simulink model "LVI_PDNN_for_QP2"  (R2020b)
settings: Solver=ode15s  StartTime=0.0  StopTime=tEnd  FixedStep=0.  MaxStep=0.2  RelTol=1e-3
values from neighbouring files (symbols this model uses):
  Ann = [-C2;         C2;         -Phi1n;         Phi1n         ]    [CreateNnMatrices.m]    (also in HvsNN.m = [-C2;     C2;     -Phi1n;     Phi1n     ]; MPC_NN.m)
  bnn = [-umin*ones(nc,1) + C1*xk(end);         umax*ones(nc,1) - C1*xk(end);         -ymin*ones(np,1) + Fn*xk + Phi2n*psiPrim;         ymax*ones(np,1) - Fn*xk - Phi2n*psiPrim         ]    [CreateNnMatrices.m]    (also in HvsNN.m = [-umin*ones(nc,1) + C1*xk(end);     umax*ones(nc,1) - C1*xk(; MPC_NN.m)
  eyenn = eye(length(Hnn))    [CreateNnMatrices.m]    (also in HvsNN.m; MPC_NN.m)
  gammann = 10000    [CreateNnMatrices.m]    (also in HvsNN.m = 0.01; MPC_NN.m = 1e+15)
  Hnn = [Wnn  -Ann'; Ann zeros(length(Ann),length(Ann'))]    [CreateNnMatrices.m]    (also in HvsNN.m; MPC_NN.m)
  nc = n_c    (= 5)    [Model_Init_Bayes.m]
  numbConstr = 3*nc + 2*np    [CreateNnMatrices.m]    (also in HvsNN.m; MPC_NN.m)
  pnn = [qnn; -bnn]    [CreateNnMatrices.m]    (also in HvsNN.m; MPC_NN.m)
  qnn = 2*((F*xk)'*W_x*Phi1 + (Phi2*psiPrim)'*W_x*Phi1)'    [CreateNnMatrices.m]    (also in HvsNN.m; MPC_NN.m)
  tEnd = 1e-2    (= 0.01)    [HvsNN.m]    (also in MPC_NN.m = 1e-07)
  Wnn = 2*(Phi1'*W_x*Phi1 + W_u)    [CreateNnMatrices.m]    (also in HvsNN.m; MPC_NN.m)
  xiM = ones(nc,1)*dumin    [CreateNnMatrices.m]    (also in HvsNN.m; MPC_NN.m = ones(nc,1)*dumin.*singleConstraint)
  xiP = ones(nc,1)*dumax    [CreateNnMatrices.m]    (also in HvsNN.m; MPC_NN.m = ones(nc,1)*dumax.*singleConstraint)
  zetaM = [xiM; bigNumber*zeros(length(Ann),1)]    [CreateNnMatrices.m]    (also in HvsNN.m; MPC_NN.m)
  zetaP = [xiP; bigNumber*ones(length(Ann),1)]    [CreateNnMatrices.m]    (also in HvsNN.m; MPC_NN.m)
undefined symbols (not defined in the file or in its folder): DiscIntNeverNeededParam, dnn, Jnn
libraries: simulink x2
settings Model: Creator=Stage  LastModifiedBy=Stage
settings SolverCC: ZeroCrossAlgorithm=Adaptive
settings DebuggingCC: IgnoredZcDiagnostic=none

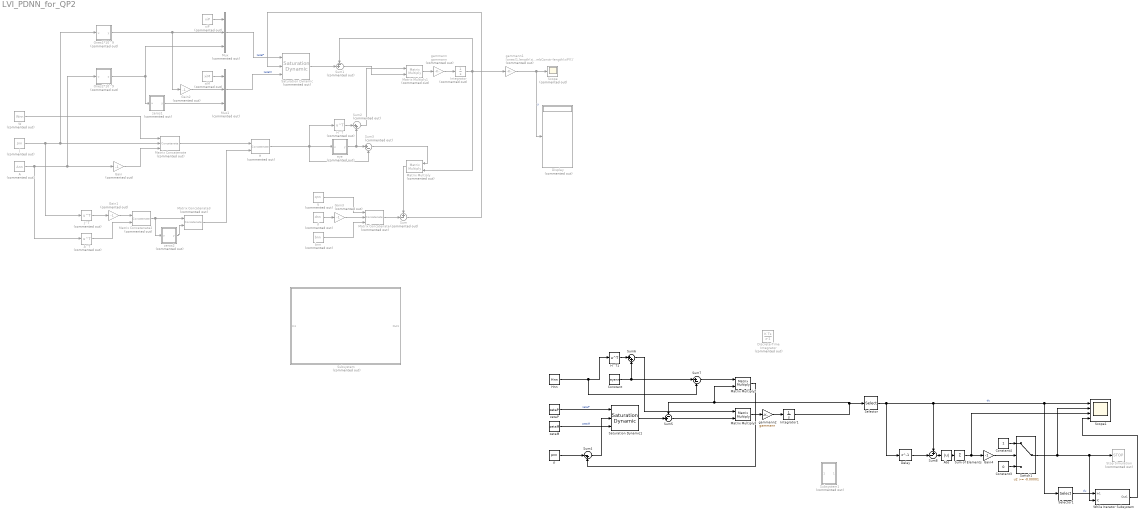
== system LVI_PDNN_for_QP2 ==
  A : Constant  Commented=on  Value=Ann
  A^T : Math  Commented=on  Operator=transpose  SaturateOnIntegerOverflow=on
  Abs : Abs
  Constant : Constant  Value=eyenn
  Constant3 : Constant  Value=0
  Constant4 : Constant
  Delay : Delay  DelayLength=1  SampleTime=tEnd/3
  Discrete-Time Integrator : DiscreteIntegrator  Commented=on  InitialCondition=0.2*(rand(numbConstr,1)-0.5)  SampleTime=0.00000000000001  ICPrevOutput=DiscIntNeverNeededParam  ICPrevScaledInput=DiscIntNeverNeededParam
  Display : Display  Commented=on
  Gain{,1..3} (4 alike) : Gain  Commented=on  Gain=-1
  Gain4 : Gain  Gain=-1
  H : Concatenate  Commented=on  Mode=Multidimensional array  ConcatenateDimension=2
  H^T : Math  Commented=on  Operator=transpose  SaturateOnIntegerOverflow=on
  H^T1 : Math  Operator=transpose  SaturateOnIntegerOverflow=on
  Hnn : Constant  Value=Hnn
  Integrator : Integrator  Commented=on  InitialCondition=0.1*(rand(numbConstr,1)-0.5)*0
  Integrator1 : Integrator  InitialCondition=.10*(rand(numbConstr,1)-0.5)
  J : Constant  Commented=on  Value=Jnn  VectorParams1D=off
  J^T : Math  Commented=on  Operator=transpose  SaturateOnIntegerOverflow=on
  Matrix Concatenate : Concatenate  Commented=on  NumInputs=3  Mode=Multidimensional array
  Matrix Concatenate2 : Concatenate  Commented=on  Mode=Multidimensional array  ConcatenateDimension=2
  Matrix Concatenate3 : Concatenate  Commented=on  Mode=Multidimensional array
  Matrix Concatenate4 : Concatenate  Commented=on  NumInputs=3  Mode=Multidimensional array
  Matrix Multiply : Product  Commented=on  Multiplication=Matrix(*)
  Matrix Multiply1 : Product  Commented=on  Multiplication=Matrix(*)
  Matrix Multiply2 : Product  Multiplication=Matrix(*)
  Matrix Multiply3 : Product  Multiplication=Matrix(*)
  Mux : Mux  Commented=on  Inputs=3
  Mux1 : Mux  Commented=on  Inputs=3
  Ones1*10^9 : MATLAB Function  Commented=on  TreatAsAtomicUnit=on
  Ones2*10^9 : MATLAB Function  Commented=on  TreatAsAtomicUnit=on
  Saturation Dynamic : simulink/Discontinuities/Saturation Dynamic  Commented=on  OutMin=[]  OutMax=[]  OutDataTypeStr=Inherit: Same as second input  OutDataType=fixdt(1, 16)  OutScaling=2^-10  DoSatur=off
  Saturation Dynamic1 : simulink/Discontinuities/Saturation Dynamic  OutMin=[]  OutMax=[]  OutDataTypeStr=Inherit: Same as second input  OutDataType=fixdt(1, 16)  OutScaling=2^-10  DoSatur=off
  Scope : Scope  Commented=on
  Scope1 : Scope  NumInputPorts=4
  Selector : Selector  InputPortWidth=numbConstr  IndexOptions=Index vector (dialog)  Indices=[1:nc]  OutputSizes=1
  Selector1 : Selector  InputPortWidth=nc  IndexOptions=Index vector (dialog)  Indices=[1]  OutputSizes=1
  Stop Simulation : Stop  Commented=on
  Subsystem : Subsystem  Commented=on
  Subsystem1 : Subsystem  Commented=on
  Sum : Sum  Commented=on  Inputs=+-|
  Sum of Elements : Sum  Inputs=+
  Sum1 : Sum  Commented=on  Inputs=-+|
  Sum2 : Sum  Commented=on  Inputs=|++
  Sum3 : Sum  Commented=on  Inputs=|+-
  Sum4 : Sum  Inputs=|-+
  Sum5 : Sum  Inputs=-+|
  Sum6 : Sum  Inputs=|++
  Sum7 : Sum  Inputs=|+-
  Sum8 : Sum  Inputs=+-|
  Switch1 : Switch  Threshold=-0.00001
  W : Constant  Commented=on  Value=Wnn
  While Iterator Subsystem : Subsystem  TreatAsAtomicUnit=on
  bnn : Constant  Commented=on  Value=bnn  VectorParams1D=off
  d : Constant  Commented=on  Value=dnn  VectorParams1D=off
  eye : MATLAB Function  Commented=on  TreatAsAtomicUnit=on
  gammann : Gain  Commented=on  Gain=gammann
  gammann1 : Gain  Commented=on  Gain=[ones(1,length(xiP)) zeros(1,numbConstr-length(xiP))]'
  gammann2 : Gain  Gain=gammann
  p : Constant  Value=pnn  VectorParams1D=off
  q : Constant  Commented=on  Value=qnn  VectorParams1D=off
  xiM : Constant  Commented=on  Value=xiM  VectorParams1D=off
  xiP : Constant  Commented=on  Value=xiP  VectorParams1D=off
  zeros1 : MATLAB Function  Commented=on  TreatAsAtomicUnit=on
  zeros2 : MATLAB Function  Commented=on  TreatAsAtomicUnit=on
  zetaM : Constant  Value=zetaM  VectorParams1D=off
  zetaP : Constant  Value=zetaP  VectorParams1D=off
  wires:
  A/1 -> A^T/1, Ones2*10^9/1(u), Gain/1
  W/1 -> Matrix Concatenate/1
  J/1 -> J^T/1, Ones1*10^9/1(u), Matrix Concatenate/2
  Gain/1 -> Matrix Concatenate/3
  Matrix Concatenate/1 -> H/1
  Matrix Concatenate2/1 -> zeros2/1(u), Matrix Concatenate3/1
  zeros2/1(y) -> Matrix Concatenate3/2
  Matrix Concatenate3/1 -> H/2
  Gain1/1 -> Matrix Concatenate2/1
  J^T/1 -> Gain1/1
  A^T/1 -> Matrix Concatenate2/2
  Ones1*10^9/1(y) -> Gain2/1, Mux/2
  xiP/1 -> Mux/1
  zeros1/1(y) -> Mux1/3
  Gain2/1 -> Mux1/2
  xiM/1 -> Mux1/1
  Mux/1 -> Saturation Dynamic/1  "zetaP"
  Mux1/1 -> Saturation Dynamic/3  "zetaM"
  d/1 -> Gain3/1
  Gain3/1 -> Matrix Concatenate4/2
  q/1 -> Matrix Concatenate4/1
  bnn/1 -> Matrix Concatenate4/3
  Matrix Concatenate4/1 -> Sum/2
  Matrix Multiply/1 -> Sum/1
  Saturation Dynamic/1 -> Sum1/2
  Matrix Multiply1/1 -> gammann/1
  gammann/1 -> Integrator/1
  H^T/1 -> Sum2/1
  Sum2/1 -> Matrix Multiply1/1
  Sum1/1 -> Matrix Multiply1/2
  H/1 -> Sum3/2, eye/1(u), H^T/1
  eye/1(y) -> Sum2/2, Sum3/1
  Sum3/1 -> Matrix Multiply/1
  Ones2*10^9/1(y) -> Mux/3, zeros1/1(u)
  Sum/1 -> Saturation Dynamic/2
  Integrator/1 -> gammann1/1, Sum1/1, Matrix Multiply/2
  gammann1/1 -> Display/1, Scope/1  "y"
  zetaM/1 -> Saturation Dynamic1/3  "zetaM"
  Matrix Multiply2/1 -> Sum4/2
  Saturation Dynamic1/1 -> Sum5/2
  Sum5/1 -> Matrix Multiply3/2
  Matrix Multiply3/1 -> gammann2/1
  zetaP/1 -> Saturation Dynamic1/1  "zetaP"
  Sum4/1 -> Saturation Dynamic1/2
  Sum7/1 -> Matrix Multiply2/1
  gammann2/1 -> Integrator1/1
  H^T1/1 -> Sum6/1
  Hnn/1 -> Sum7/2, H^T1/1
  p/1 -> Sum4/1
  Constant/1 -> Sum6/2, Sum7/1
  Sum6/1 -> Matrix Multiply3/1
  Integrator1/1 -> Matrix Multiply2/2, Sum5/1, Selector/1
  Selector/1 -> Delay/1, Sum8/1, Selector1/1, Scope1/1  "du"
  Delay/1 -> Sum8/2
  Constant4/1 -> Switch1/1
  Constant3/1 -> Switch1/3
  Switch1/1 -> While Iterator Subsystem/2(IC), Stop Simulation/1, Scope1/2
  Sum of Elements/1 -> Gain4/1, Scope1/3
  Gain4/1 -> Switch1/2
  Sum8/1 -> Abs/1
  Abs/1 -> Sum of Elements/1
  Selector1/1 -> While Iterator Subsystem/1(In1)  "du"
  While Iterator Subsystem/1(Out1) -> Scope1/4

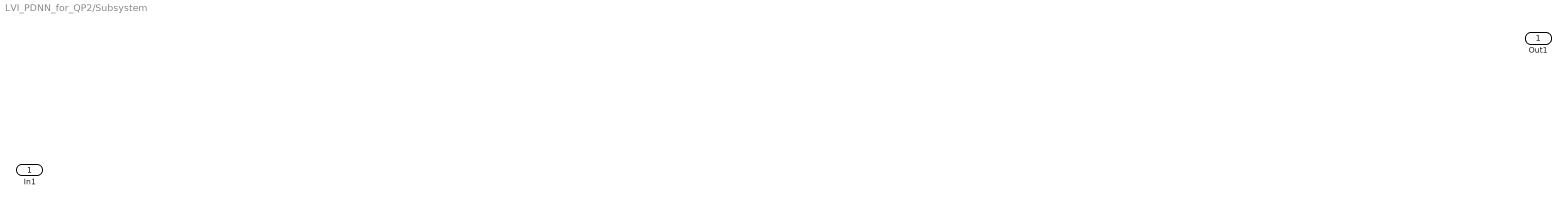
== system LVI_PDNN_for_QP2/Subsystem ==
  In1 : Inport
  Out1 : Outport

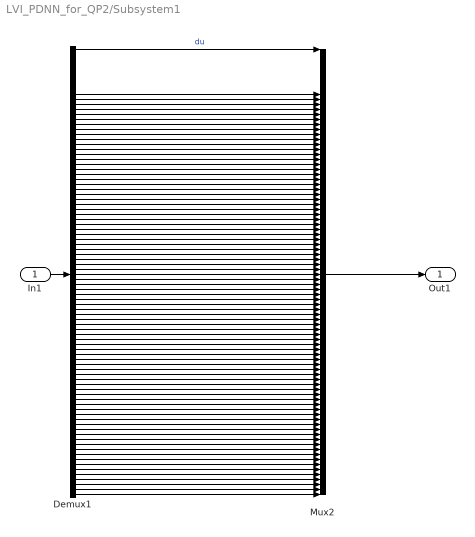
== system LVI_PDNN_for_QP2/Subsystem1 ==
  In1 : Inport
  Demux1 : Demux  Outputs=numbConstr
  Mux2 : Mux  Inputs=numbConstr
  Out1 : Outport
  wires:
  Demux1/11 -> Mux2/11
  Demux1/37 -> Mux2/37
  Demux1/80 -> Mux2/80
  Demux1/16 -> Mux2/16
  Demux1/46 -> Mux2/46
  Demux1/58 -> Mux2/58
  Demux1/40 -> Mux2/40
  Demux1/31 -> Mux2/31
  Demux1/12 -> Mux2/12
  Demux1/1 -> Mux2/1  "du"
  Demux1/28 -> Mux2/28
  Demux1/67 -> Mux2/67
  Demux1/69 -> Mux2/69
  Demux1/26 -> Mux2/26
  Demux1/17 -> Mux2/17
  Demux1/73 -> Mux2/73
  Demux1/53 -> Mux2/53
  Demux1/14 -> Mux2/14
  Demux1/34 -> Mux2/34
  Demux1/24 -> Mux2/24
  Demux1/76 -> Mux2/76
  Demux1/49 -> Mux2/49
  Demux1/88 -> Mux2/88
  Demux1/57 -> Mux2/57
  Demux1/39 -> Mux2/39
  Demux1/15 -> Mux2/15
  Demux1/54 -> Mux2/54
  Demux1/77 -> Mux2/77
  Demux1/72 -> Mux2/72
  Demux1/36 -> Mux2/36
  Demux1/60 -> Mux2/60
  Demux1/66 -> Mux2/66
  Demux1/29 -> Mux2/29
  Demux1/42 -> Mux2/42
  Demux1/87 -> Mux2/87
  Demux1/32 -> Mux2/32
  Demux1/78 -> Mux2/78
  Demux1/90 -> Mux2/90
  Demux1/22 -> Mux2/22
  Demux1/10 -> Mux2/10
  Demux1/13 -> Mux2/13
  Demux1/62 -> Mux2/62
  Demux1/89 -> Mux2/89
  Demux1/35 -> Mux2/35
  Demux1/23 -> Mux2/23
  Demux1/41 -> Mux2/41
  Demux1/30 -> Mux2/30
  Demux1/48 -> Mux2/48
  Demux1/47 -> Mux2/47
  Demux1/51 -> Mux2/51
  Demux1/43 -> Mux2/43
  Demux1/52 -> Mux2/52
  Demux1/74 -> Mux2/74
  Demux1/70 -> Mux2/70
  Demux1/19 -> Mux2/19
  Demux1/33 -> Mux2/33
  Demux1/68 -> Mux2/68
  Demux1/20 -> Mux2/20
  Demux1/59 -> Mux2/59
  Demux1/85 -> Mux2/85
  Demux1/65 -> Mux2/65
  Demux1/21 -> Mux2/21
  Demux1/50 -> Mux2/50
  Demux1/38 -> Mux2/38
  Demux1/82 -> Mux2/82
  Demux1/81 -> Mux2/81
  Demux1/55 -> Mux2/55
  Demux1/71 -> Mux2/71
  Demux1/86 -> Mux2/86
  Demux1/25 -> Mux2/25
  Demux1/45 -> Mux2/45
  Demux1/44 -> Mux2/44
  Demux1/18 -> Mux2/18
  Demux1/63 -> Mux2/63
  Demux1/83 -> Mux2/83
  Demux1/84 -> Mux2/84
  Demux1/56 -> Mux2/56
  Demux1/64 -> Mux2/64
  In1/1 -> Demux1/1
  Demux1/75 -> Mux2/75
  Demux1/27 -> Mux2/27
  Demux1/79 -> Mux2/79
  Demux1/61 -> Mux2/61
  Mux2/1 -> Out1/1

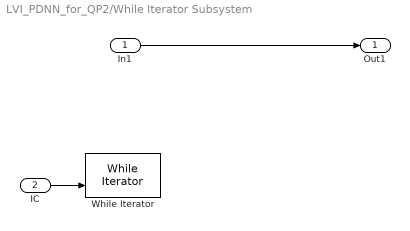
== system LVI_PDNN_for_QP2/While Iterator Subsystem ==
  In1 : Inport
  IC : Inport  Port=2
  While Iterator : WhileIterator
  Out1 : Outport
  wires:
  IC/1 -> While Iterator/2
  In1/1 -> Out1/1

== matlab function LVI_PDNN_for_QP2/zeros2 ==
  data: u input; y output
function y = fcn(u)

    asd = size(u);
    


y = zeros(asd(2),asd(2));

== matlab function LVI_PDNN_for_QP2/Ones2*10^9 ==
  data: u input; y output
function y = fcn(u)
asd = size(u);
y = ones(asd(1),1)*10^6;

== matlab function LVI_PDNN_for_QP2/eye ==
  data: u input; y output
    function y = fcn(u)

       


y = eye(length(u));

== matlab function LVI_PDNN_for_QP2/zeros1 ==
  data: u input; y output
function y = fcn(u)

asd = size(u);
y = zeros(length(u),1);

== matlab function LVI_PDNN_for_QP2/Ones1*10^9 ==
  data: u input; y output
function y = fcn(u)
asd = size(u);
y = ones(asd(1),1)*10^6;
